simulink library "UtilsLib"  (Simulink 7.7)
settings: Solver=ode45  SolverMode=SingleTasking  StartTime=0.0  StopTime=10.0  RelTol=1e-3
undefined symbols (not defined in the file or in its folder): gca, get, hot, magnitude, Newton, Raphson
libraries: simulink x13, dspsigattribs x2, dspsnks4 x1, dspstat3 x1, UtilsLib x1
settings Model: Creator=jpalma  LastModifiedBy=jpalma

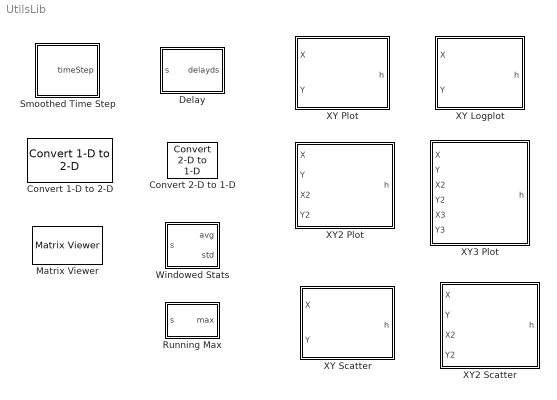
== system UtilsLib ==
  Convert 1-D to 2-D : dspsigattribs/Convert 1-D to 2-D  SystemSampleTime=-1  M=1  N=1  frameBasedOut=off
  Convert 2-D to 1-D : dspsigattribs/Convert 2-D to 1-D  SystemSampleTime=-1
  Delay : Subsystem  mask{Delay=1, IC=0}
      mask prompts: IC "Initial Output"
  Matrix Viewer : dspsnks4/Matrix Viewer  ImageParams=off  CMapStr=hot(256)  AxisColorbar=on  AxisParams=off  AxisOrigin=Upper left corner  XLabel=X-axis  YLabel=Y-axis  ZLabel=Z-axis  FigPos=get(0,'defaultfigureposition')  AxisZoom=off
      settings: YMin=-1.0  YMax=1.0
  Running Max : Subsystem  mask{IC=0}
      mask prompts: IC "Initial Value"
  Smoothed Time Step : Subsystem  mask{timeStepsSmoothed=10}
      mask prompts: timeStepsSmoothed "Number of Time Steps Smoothed"
      mask help:
      | What are the time units?
      | Author: Jesse Palma
      mask Help: Author: Jesse Palma
      mask Display: image(imread('../Libs/icons/TimeStep.JPG'), 'center');
  Windowed Stats : Subsystem  mask{winL=100}
      mask prompts: winL "Window Size"
      mask help:
      | Computes avg (arithematic mean) and standard deviation (std, sqrt of variance) over a specific window
      |
      | Block Authors: Jesse Palma and Himanshu Mhatre
      mask Help:
      | Computes avg (arithematic mean) and standard deviation (std, sqrt of variance) over a specific window
      | 
      | Block Authors: Jesse Palma and Himanshu Mhatre
  XY Logplot : Subsystem  mask{plotInt=10}
      mask prompts: plotInt "Plotting Interval (Sim steps)"
      mask help: Author: Jesse Palma
      mask Help: Author: Jesse Palma
      mask Display: image(imread('../Libs/icons/XYFunc.JPG'),'center');
  XY Plot : Subsystem  mask{plotInt=10}
      mask prompts: plotInt "Plotting Interval (Sim steps)"
      mask help: Author: Jesse Palma
      mask Help: Author: Jesse Palma
      mask Display: image(imread('../Libs/icons/XYFunc.JPG'),'center');
  XY Scatter : Subsystem  mask{plotInt=10}
      mask prompts: plotInt "Plotting Interval (Sim steps)"
      mask help: Author: Jesse Palma
      mask Help: Author: Jesse Palma
      mask Display: image(imread('../Libs/icons/XYFunc.JPG'),'center');
  XY2 Plot : Subsystem  mask{plotInt=10}
      mask prompts: plotInt "Plotting Interval (Sim steps)"
      mask help: Author: Jesse Palma
      mask Help: Author: Jesse Palma
      mask Display: image(imread('../Libs/icons/XYFunc.JPG'),'center');
  XY2 Scatter : Subsystem  mask{plotInt=10}
      mask prompts: plotInt "Plotting Interval (Sim steps)"
      mask help: Author: Jesse Palma
      mask Help: Author: Jesse Palma
      mask Display: image(imread('../Libs/icons/XYFunc.JPG'),'center');
  XY3 Plot : Subsystem  mask{plotInt=10}
      mask prompts: plotInt "Plotting Interval (Sim steps)"
      mask help: Author: Jesse Palma
      mask Help: Author: Jesse Palma
      mask Display: image(imread('../Libs/icons/XYFunc.JPG'),'center');

== system UtilsLib/Delay ==
  s : Inport
  Transport Delay : TransportDelay  DelayTime=Delay  InitialOutput=IC
  delayds : Outport
  wires:
  s/1 -> Transport Delay/1
  Transport Delay/1 -> delayds/1

== system UtilsLib/Running Max ==
  s : Inport
  Memory : Memory  X0=IC
  MinMax : MinMax  Function=max  Inputs=2
  max : Outport
  wires:
  s/1 -> MinMax/1
  Memory/1 -> MinMax/2
  MinMax/1 -> max/1, Memory/1

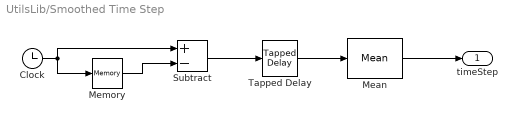
== system UtilsLib/Smoothed Time Step ==
  Clock : Clock
      settings: Decimation=10
  Mean : dspstat3/Mean  run=off  reset_popup=None  directionMode=Each column  dimension=1  treatSBRowAsCol=on  roiEnable=off  roiType=Rectangles  roiPortion=Entire ROI  roiOutput=Individual statistics for each ROI  roiFlag=off  outputDataTypeStr=Inherit: Same as accumulator  outputLastDataTypeStr=Inherit: Same as accumulator  outputMin=[]  outputMax=[]  roundingMode=Floor  overflowMode=off
  Memory : Memory
  Subtract : Sum  Inputs=+-
  Tapped Delay : simulink/Discrete/Tapped Delay  vinit=0  samptime=-1  NumDelays=timeStepsSmoothed  DelayOrder=Oldest  includeCurrent=off
  timeStep : Outport
  wires:
  Clock/1 -> Memory/1, Subtract/1
  Memory/1 -> Subtract/2
  Subtract/1 -> Tapped Delay/1
  Tapped Delay/1 -> Mean/1
  Mean/1 -> timeStep/1

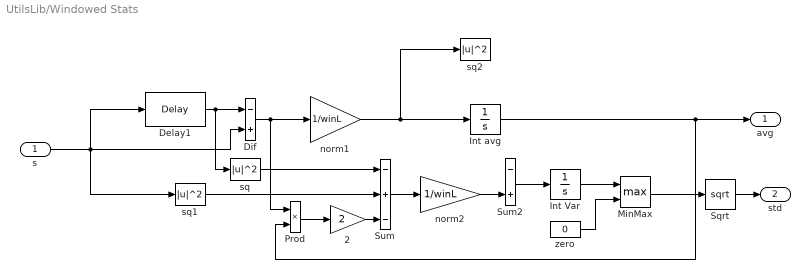
== system UtilsLib/Windowed Stats ==
  s : Inport
  2 : Gain  Gain=2
  Delay1 : UtilsLib/Delay  SystemSampleTime=-1  Delay=winL  IC=0
  Dif : Sum  Inputs=-+
  Int Var : Integrator  LowerSaturationLimit=0
  Int avg : Integrator
  MinMax : MinMax  Function=max  Inputs=2
  Prod : Product  Inputs=**
  Sqrt : Sqrt  AlgorithmType=Newton-Raphson  SaturateOnIntegerOverflow=on
  Sum : Sum  Inputs=-+-
  Sum2 : Sum  Inputs=-+
  norm1 : Gain  Gain=1/winL
  norm2 : Gain  Gain=1/winL
  sq : Math  Operator=magnitude^2  SaturateOnIntegerOverflow=on
  sq1 : Math  Operator=magnitude^2  SaturateOnIntegerOverflow=on
  sq2 : Math  Operator=magnitude^2  SaturateOnIntegerOverflow=on
  zero : Constant  Value=0
  avg : Outport
  std : Outport  Port=2
  wires:
  norm2/1 -> Sum2/2
  norm1/1 -> Int avg/1, sq2/1
  Delay1/1 -> Dif/1, sq/1
  Dif/1 -> norm1/1, Prod/1
  sq/1 -> Sum/1
  sq1/1 -> Sum/2
  Int avg/1 -> Prod/2, avg/1
  Prod/1 -> 2/1
  2/1 -> Sum/3
  Sum/1 -> norm2/1
  Sum2/1 -> Int Var/1
  Sqrt/1 -> std/1
  s/1 -> Delay1/1, sq1/1, Dif/2
  Int Var/1 -> MinMax/1
  zero/1 -> MinMax/2
  MinMax/1 -> Sqrt/1

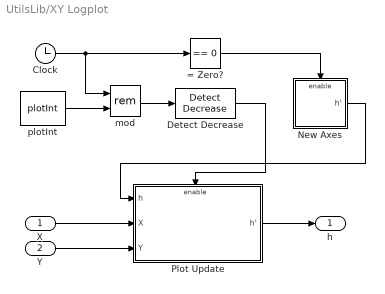
== system UtilsLib/XY Logplot ==
  X : Inport
  Y : Inport  Port=2
  = Zero? : simulink/Logic and Bit Operations/Compare To Zero  SystemSampleTime=-1  relop===  LogicOutDataTypeMode=uint8
  Clock : Clock
      settings: Decimation=10
  Detect Decrease : simulink/Logic and Bit Operations/Detect Decrease  SystemSampleTime=-1  vinit=0.0
  New Axes : Subsystem
  Plot Update : Subsystem
  mod : Math  Operator=rem  SaturateOnIntegerOverflow=on
  plotInt : Constant  Value=plotInt
  h : Outport
  wires:
  Detect Decrease/1 -> Plot Update/Enable
  New Axes/1(h') -> Plot Update/1(h)
  = Zero?/1 -> New Axes/Enable
  mod/1 -> Detect Decrease/1
  Clock/1 -> = Zero?/1, mod/1
  plotInt/1 -> mod/2
  Y/1 -> Plot Update/3(Y)
  Plot Update/1(h') -> h/1
  X/1 -> Plot Update/2(X)

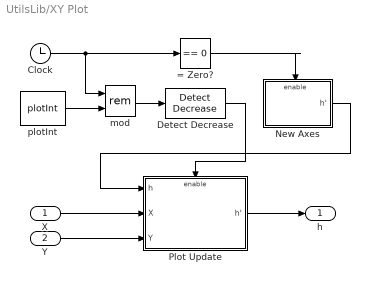
== system UtilsLib/XY Plot ==
  X : Inport
  Y : Inport  Port=2
  = Zero? : simulink/Logic and Bit Operations/Compare To Zero  SystemSampleTime=-1  relop===  LogicOutDataTypeMode=uint8
  Clock : Clock
      settings: Decimation=10
  Detect Decrease : simulink/Logic and Bit Operations/Detect Decrease  SystemSampleTime=-1  vinit=0.0
  New Axes : Subsystem
  Plot Update : Subsystem
  mod : Math  Operator=rem  SaturateOnIntegerOverflow=on
  plotInt : Constant  Value=plotInt
  h : Outport
  wires:
  X/1 -> Plot Update/2(X)
  Plot Update/1(h') -> h/1
  Y/1 -> Plot Update/3(Y)
  plotInt/1 -> mod/2
  Clock/1 -> mod/1, = Zero?/1
  mod/1 -> Detect Decrease/1
  = Zero?/1 -> New Axes/Enable
  New Axes/1(h') -> Plot Update/1(h)
  Detect Decrease/1 -> Plot Update/Enable

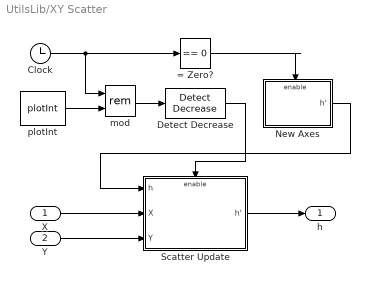
== system UtilsLib/XY Scatter ==
  X : Inport
  Y : Inport  Port=2
  = Zero? : simulink/Logic and Bit Operations/Compare To Zero  SystemSampleTime=-1  relop===  LogicOutDataTypeMode=uint8
  Clock : Clock
      settings: Decimation=10
  Detect Decrease : simulink/Logic and Bit Operations/Detect Decrease  SystemSampleTime=-1  vinit=0.0
  New Axes : Subsystem
  Scatter Update : Subsystem
  mod : Math  Operator=rem  SaturateOnIntegerOverflow=on
  plotInt : Constant  Value=plotInt
  h : Outport
  wires:
  Detect Decrease/1 -> Scatter Update/Enable
  New Axes/1(h') -> Scatter Update/1(h)
  = Zero?/1 -> New Axes/Enable
  mod/1 -> Detect Decrease/1
  Clock/1 -> = Zero?/1, mod/1
  plotInt/1 -> mod/2
  Y/1 -> Scatter Update/3(Y)
  Scatter Update/1(h') -> h/1
  X/1 -> Scatter Update/2(X)

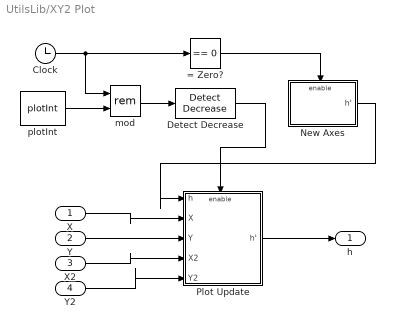
== system UtilsLib/XY2 Plot ==
  X : Inport
  Y : Inport  Port=2
  X2 : Inport  Port=3
  Y2 : Inport  Port=4
  = Zero? : simulink/Logic and Bit Operations/Compare To Zero  SystemSampleTime=-1  relop===  LogicOutDataTypeMode=uint8
  Clock : Clock
      settings: Decimation=10
  Detect Decrease : simulink/Logic and Bit Operations/Detect Decrease  SystemSampleTime=-1  vinit=0.0
  New Axes : Subsystem
  Plot Update : Subsystem
  mod : Math  Operator=rem  SaturateOnIntegerOverflow=on
  plotInt : Constant  Value=plotInt
  h : Outport
  wires:
  Detect Decrease/1 -> Plot Update/Enable
  New Axes/1(h') -> Plot Update/1(h)
  = Zero?/1 -> New Axes/Enable
  mod/1 -> Detect Decrease/1
  Clock/1 -> = Zero?/1, mod/1
  plotInt/1 -> mod/2
  Y/1 -> Plot Update/3(Y)
  Plot Update/1(h') -> h/1
  X/1 -> Plot Update/2(X)
  X2/1 -> Plot Update/4(X2)
  Y2/1 -> Plot Update/5(Y2)

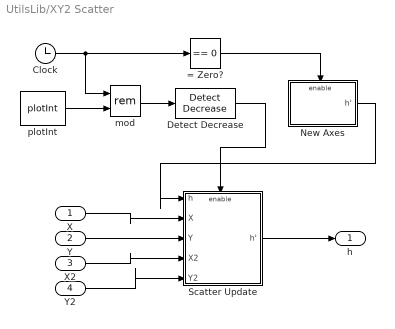
== system UtilsLib/XY2 Scatter ==
  X : Inport
  Y : Inport  Port=2
  X2 : Inport  Port=3
  Y2 : Inport  Port=4
  = Zero? : simulink/Logic and Bit Operations/Compare To Zero  SystemSampleTime=-1  relop===  LogicOutDataTypeMode=uint8
  Clock : Clock
      settings: Decimation=10
  Detect Decrease : simulink/Logic and Bit Operations/Detect Decrease  SystemSampleTime=-1  vinit=0.0
  New Axes : Subsystem
  Scatter Update : Subsystem
  mod : Math  Operator=rem  SaturateOnIntegerOverflow=on
  plotInt : Constant  Value=plotInt
  h : Outport
  wires:
  Y2/1 -> Scatter Update/5(Y2)
  X2/1 -> Scatter Update/4(X2)
  X/1 -> Scatter Update/2(X)
  Scatter Update/1(h') -> h/1
  Y/1 -> Scatter Update/3(Y)
  plotInt/1 -> mod/2
  Clock/1 -> mod/1, = Zero?/1
  mod/1 -> Detect Decrease/1
  = Zero?/1 -> New Axes/Enable
  New Axes/1(h') -> Scatter Update/1(h)
  Detect Decrease/1 -> Scatter Update/Enable

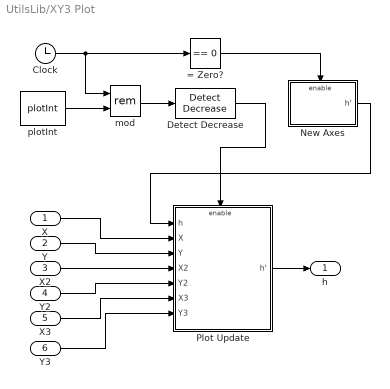
== system UtilsLib/XY3 Plot ==
  X : Inport
  Y : Inport  Port=2
  X2 : Inport  Port=3
  Y2 : Inport  Port=4
  X3 : Inport  Port=5
  Y3 : Inport  Port=6
  = Zero? : simulink/Logic and Bit Operations/Compare To Zero  SystemSampleTime=-1  relop===  LogicOutDataTypeMode=uint8
  Clock : Clock
      settings: Decimation=10
  Detect Decrease : simulink/Logic and Bit Operations/Detect Decrease  SystemSampleTime=-1  vinit=0.0
  New Axes : Subsystem
  Plot Update : Subsystem
  mod : Math  Operator=rem  SaturateOnIntegerOverflow=on
  plotInt : Constant  Value=plotInt
  h : Outport
  wires:
  Y2/1 -> Plot Update/5(Y2)
  X2/1 -> Plot Update/4(X2)
  X/1 -> Plot Update/2(X)
  Plot Update/1(h') -> h/1
  Y/1 -> Plot Update/3(Y)
  plotInt/1 -> mod/2
  Clock/1 -> mod/1, = Zero?/1
  mod/1 -> Detect Decrease/1
  = Zero?/1 -> New Axes/Enable
  Detect Decrease/1 -> Plot Update/Enable
  New Axes/1(h') -> Plot Update/1(h)
  X3/1 -> Plot Update/6(X3)
  Y3/1 -> Plot Update/7(Y3)

== system UtilsLib/XY Logplot/New Axes ==
  Enable : EnablePort
  Axes : MATLABFcn  MATLABFcn=gca;
  fig : MATLABFcn  MATLABFcn=figure();
  h' : Outport
  wires:
  Axes/1 -> h'/1
  fig/1 -> Axes/1

== system UtilsLib/XY Logplot/Plot Update ==
  h : Inport
  X : Inport  Port=2
  Y : Inport  Port=3
  Enable : EnablePort
  L2 M-file S-Funct : M-S-Function  FunctionName=SLogPlot
  h' : Outport
  wires:
  L2 M-file S-Funct/1 -> h'/1
  Y/1 -> L2 M-file S-Funct/3
  X/1 -> L2 M-file S-Funct/2
  h/1 -> L2 M-file S-Funct/1

== system UtilsLib/XY Plot/New Axes ==
  Enable : EnablePort
  Axes : MATLABFcn  MATLABFcn=gca;
  fig : MATLABFcn  MATLABFcn=figure();
  h' : Outport
  wires:
  Axes/1 -> h'/1
  fig/1 -> Axes/1

== system UtilsLib/XY Plot/Plot Update ==
  h : Inport
  X : Inport  Port=2
  Y : Inport  Port=3
  Enable : EnablePort
  L2 M-file S-Funct : M-S-Function  FunctionName=SPlot
  h' : Outport
  wires:
  h/1 -> L2 M-file S-Funct/1
  X/1 -> L2 M-file S-Funct/2
  Y/1 -> L2 M-file S-Funct/3
  L2 M-file S-Funct/1 -> h'/1

== system UtilsLib/XY Scatter/New Axes ==
  Enable : EnablePort
  Axes : MATLABFcn  MATLABFcn=gca;
  fig : MATLABFcn  MATLABFcn=figure();
  h' : Outport
  wires:
  fig/1 -> Axes/1
  Axes/1 -> h'/1

== system UtilsLib/XY Scatter/Scatter Update ==
  h : Inport
  X : Inport  Port=2
  Y : Inport  Port=3
  Enable : EnablePort
  L2 M-file S-Funct : M-S-Function  FunctionName=SScatter
  h' : Outport
  wires:
  L2 M-file S-Funct/1 -> h'/1
  Y/1 -> L2 M-file S-Funct/3
  X/1 -> L2 M-file S-Funct/2
  h/1 -> L2 M-file S-Funct/1

== system UtilsLib/XY2 Plot/New Axes ==
  Enable : EnablePort
  Axes : MATLABFcn  MATLABFcn=gca();
  fig : MATLABFcn  MATLABFcn=figure();
  h' : Outport
  wires:
  Axes/1 -> h'/1
  fig/1 -> Axes/1

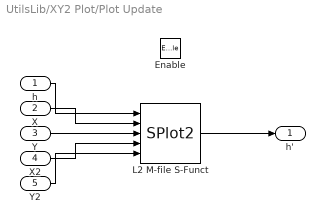
== system UtilsLib/XY2 Plot/Plot Update ==
  h : Inport
  X : Inport  Port=2
  Y : Inport  Port=3
  X2 : Inport  Port=4
  Y2 : Inport  Port=5
  Enable : EnablePort
  L2 M-file S-Funct : M-S-Function  FunctionName=SPlot2
  h' : Outport
  wires:
  L2 M-file S-Funct/1 -> h'/1
  Y/1 -> L2 M-file S-Funct/3
  X/1 -> L2 M-file S-Funct/2
  h/1 -> L2 M-file S-Funct/1
  X2/1 -> L2 M-file S-Funct/4
  Y2/1 -> L2 M-file S-Funct/5

== system UtilsLib/XY2 Scatter/New Axes ==
  Enable : EnablePort
  Axes : MATLABFcn  MATLABFcn=gca();
  fig : MATLABFcn  MATLABFcn=figure();
  h' : Outport
  wires:
  fig/1 -> Axes/1
  Axes/1 -> h'/1

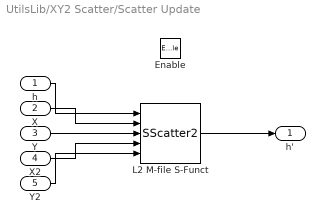
== system UtilsLib/XY2 Scatter/Scatter Update ==
  h : Inport
  X : Inport  Port=2
  Y : Inport  Port=3
  X2 : Inport  Port=4
  Y2 : Inport  Port=5
  Enable : EnablePort
  L2 M-file S-Funct : M-S-Function  FunctionName=SScatter2
  h' : Outport
  wires:
  Y2/1 -> L2 M-file S-Funct/5
  X2/1 -> L2 M-file S-Funct/4
  h/1 -> L2 M-file S-Funct/1
  X/1 -> L2 M-file S-Funct/2
  Y/1 -> L2 M-file S-Funct/3
  L2 M-file S-Funct/1 -> h'/1

== system UtilsLib/XY3 Plot/New Axes ==
  Enable : EnablePort
  Axes : MATLABFcn  MATLABFcn=gca;
  Fig : MATLABFcn  MATLABFcn=figure();
  h' : Outport
  wires:
  Axes/1 -> h'/1
  Fig/1 -> Axes/1

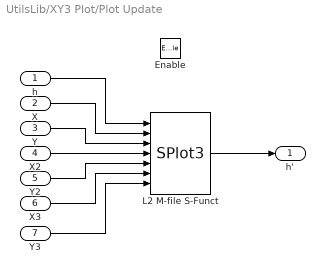
== system UtilsLib/XY3 Plot/Plot Update ==
  h : Inport
  X : Inport  Port=2
  Y : Inport  Port=3
  X2 : Inport  Port=4
  Y2 : Inport  Port=5
  X3 : Inport  Port=6
  Y3 : Inport  Port=7
  Enable : EnablePort
  L2 M-file S-Funct : M-S-Function  FunctionName=SPlot3
  h' : Outport
  wires:
  Y2/1 -> L2 M-file S-Funct/5
  X2/1 -> L2 M-file S-Funct/4
  h/1 -> L2 M-file S-Funct/1
  X/1 -> L2 M-file S-Funct/2
  Y/1 -> L2 M-file S-Funct/3
  L2 M-file S-Funct/1 -> h'/1
  X3/1 -> L2 M-file S-Funct/6
  Y3/1 -> L2 M-file S-Funct/7
